simulink model "Problem5"  (R2020b)
settings: Solver=VariableStepAuto  StartTime=0.0  StopTime=10.0  RelTol=1e-3
values from neighbouring files (symbols this model uses):
  C = 0.00001    (= 1e-05)    [parameters.m]
  R = 10    [parameters.m]
settings Model: Creator=adity  LastModifiedBy=adity

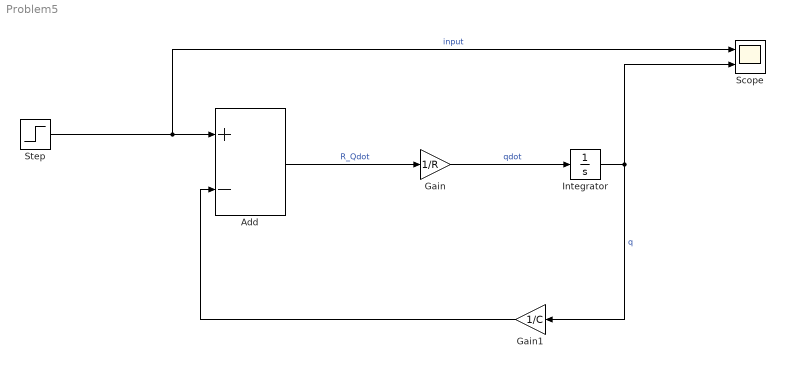
== system Problem5 ==
  Add : Sum  Inputs=+-
  Gain : Gain  Gain=1/R
  Gain1 : Gain  Gain=1/C
  Integrator : Integrator  InitialCondition=2
  Scope : Scope  NumInputPorts=2
  Step : Step  SampleTime=0
  wires:
  Gain1/1 -> Add/2
  Step/1 -> Scope/1, Add/1  "input"
  Gain/1 -> Integrator/1  "qdot"
  Integrator/1 -> Gain1/1, Scope/2  "q"
  Add/1 -> Gain/1  "R_Qdot"
